simulink model "aircraft_trimLin"  (R2023a)
settings: Solver=VariableStepAuto  StartTime=0.0  StopTime=TF  RelTol=1e-3
values from neighbouring files (symbols this model uses):
  x0 = [85; 0; 0; 0; 0; 0; 0; 0.1; 0; 44.94028*pi/180; -73.09747*pi/180; 3000*0.2808]    [init.m]
undefined symbols (not defined in the file or in its folder): aircraft_6DOF_model
libraries: aerolibfltsims x2, aerolibanimutils x1
settings Model: Creator=Hegde  LastModifiedBy=Hegde

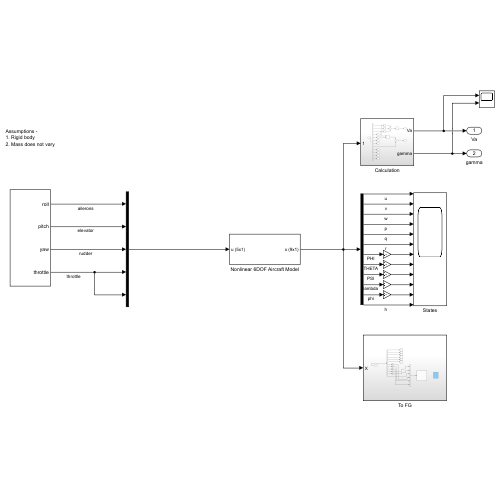
[thumbnail: Simulink's stored preview of the top-level diagram]
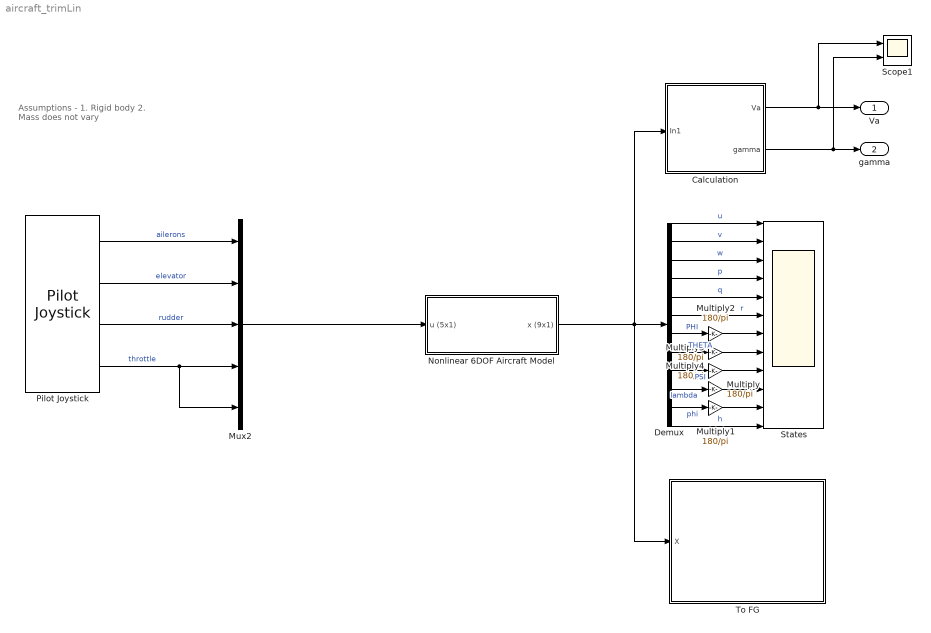
== system aircraft_trimLin ==
  note: Assumptions -
      | 1. Rigid body
      | 2. Mass does not vary
  Calculation : Subsystem
  Demux : Demux  Outputs=12
  Multiply{,1..4} (5 alike) : Gain  Gain=180/pi
  Mux2 : Mux  Inputs=5
  Nonlinear 6DOF Aircraft Model : Subsystem
  Pilot Joystick : aerolibanimutils/Pilot Joystick  JoystickID=Joystick1  OutputConfiguration=FourAxis  SampleTime=1/30
  Scope1 : Scope  NumInputPorts=2
  States : Scope  NumInputPorts=12
  To FG : Subsystem
  Va : Outport
  gamma : Outport  Port=2
  wires:
  Demux/1 -> States/1  "u"
  Demux/2 -> States/2  "v"
  Demux/3 -> States/3  "w"
  Demux/4 -> States/4  "p"
  Demux/5 -> States/5  "q"
  Demux/6 -> States/6  "r"
  Demux/7 -> Multiply2/1  "PHI"
  Demux/8 -> Multiply3/1  "THETA"
  Demux/9 -> Multiply4/1  "PSI"
  Calculation/2(gamma) -> Scope1/2, gamma/1
  Calculation/1(Va) -> Va/1, Scope1/1
  Mux2/1 -> Nonlinear 6DOF Aircraft Model/1(u (5x1))
  Pilot Joystick/1 -> Mux2/1  "ailerons"
  Pilot Joystick/2 -> Mux2/2  "elevator"
  Pilot Joystick/3 -> Mux2/3  "rudder"
  Pilot Joystick/4 -> Mux2/4, Mux2/5  "throttle"
  Demux/10 -> Multiply/1  "lambda"
  Demux/11 -> Multiply1/1  "phi"
  Demux/12 -> States/12  "h"
  Multiply/1 -> States/10
  Multiply1/1 -> States/11
  Multiply2/1 -> States/7
  Multiply3/1 -> States/8
  Multiply4/1 -> States/9
  Nonlinear 6DOF Aircraft Model/1(x (9x1)) -> To FG/1(X), Demux/1, Calculation/1(In1)

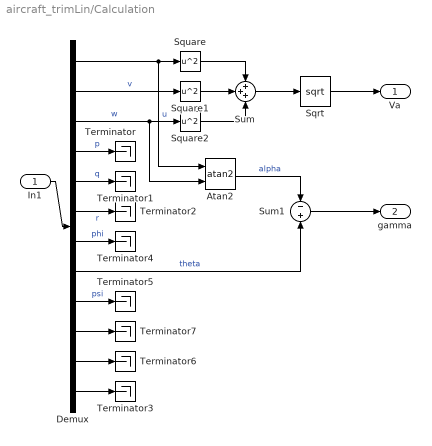
== system aircraft_trimLin/Calculation ==
  In1 : Inport
  Atan2 : Trigonometry  Operator=atan2
  Demux : Demux  Outputs=12
  Sqrt : Sqrt
  Square : Math  Operator=square
  Square1 : Math  Operator=square
  Square2 : Math  Operator=square
  Sum : Sum  Inputs=+++
  Sum1 : Sum  Inputs=-+
  Terminator{,1..7} (8 alike) : Terminator
  Va : Outport
  gamma : Outport  Port=2
  wires:
  Demux/1 -> Atan2/1, Square/1  "u"
  Square/1 -> Sum/1
  Demux/9 -> Terminator5/1  "psi"
  Demux/5 -> Terminator1/1  "q"
  Demux/3 -> Square2/1, Atan2/2  "w"
  In1/1 -> Demux/1
  Demux/2 -> Square1/1  "v"
  Demux/6 -> Terminator2/1  "r"
  Atan2/1 -> Sum1/1  "alpha"
  Demux/4 -> Terminator/1  "p"
  Sum1/1 -> gamma/1
  Square2/1 -> Sum/3
  Sum/1 -> Sqrt/1
  Demux/7 -> Terminator4/1  "phi"
  Demux/8 -> Sum1/2  "theta"
  Square1/1 -> Sum/2
  Sqrt/1 -> Va/1
  Demux/12 -> Terminator3/1
  Demux/10 -> Terminator7/1
  Demux/11 -> Terminator6/1

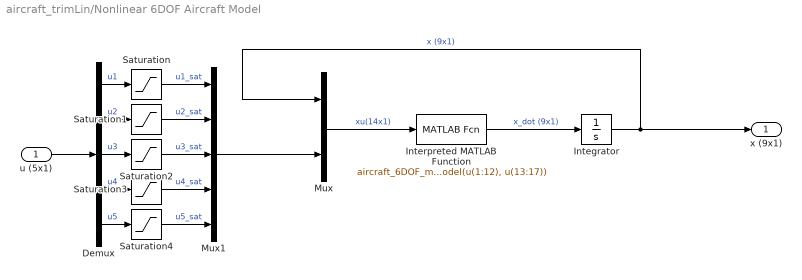
== system aircraft_trimLin/Nonlinear 6DOF Aircraft Model ==
  u (5x1) : Inport
  Demux : Demux  Outputs=5
  Integrator : Integrator  InitialCondition=x0
  Interpreted MATLAB Function : MATLABFcn  MATLABFcn=aircraft_6DOF_model(u(1:12), u(13:17))
  Mux : Mux  Inputs=2
  Mux1 : Mux  Inputs=5
  Saturation : Saturate  UpperLimit=25 * pi/180  LowerLimit=-25 * pi/180
  Saturation1 : Saturate  UpperLimit=10 * pi/180  LowerLimit=-25 * pi/180
  Saturation2 : Saturate  UpperLimit=30 * pi/180  LowerLimit=-30 * pi/180
  Saturation3 : Saturate  UpperLimit=1  LowerLimit=0
  Saturation4 : Saturate  UpperLimit=1  LowerLimit=0
  x (9x1) : Outport
  wires:
  Integrator/1 -> x (9x1)/1, Mux/1  "x (9x1)"
  Interpreted MATLAB Function/1 -> Integrator/1  "x_dot (9x1)"
  Mux/1 -> Interpreted MATLAB Function/1  "xu(14x1)"
  u (5x1)/1 -> Demux/1
  Demux/1 -> Saturation/1  "u1"
  Saturation/1 -> Mux1/1  "u1_sat"
  Demux/2 -> Saturation1/1  "u2"
  Saturation1/1 -> Mux1/2  "u2_sat"
  Demux/3 -> Saturation2/1  "u3"
  Saturation2/1 -> Mux1/3  "u3_sat"
  Demux/4 -> Saturation3/1  "u4"
  Demux/5 -> Saturation4/1  "u5"
  Saturation3/1 -> Mux1/4  "u4_sat"
  Saturation4/1 -> Mux1/5  "u5_sat"
  Mux1/1 -> Mux/2

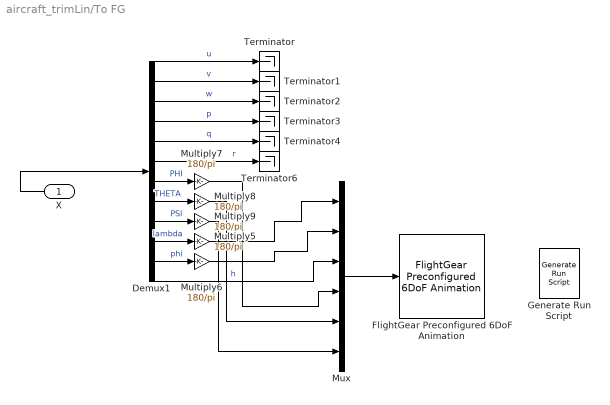
== system aircraft_trimLin/To FG ==
  X : Inport
  Demux1 : Demux  Outputs=12
  FlightGear Preconfigured 6DoF Animation : aerolibfltsims/FlightGear Preconfigured 6DoF Animation  xFlightGearVersion=v2019.1  DestinationIpAddress=127.0.0.1  DestinationPort=5502  SampleTime=1/30  packetVersion=24
  Generate Run Script : aerolibfltsims/Generate Run Script  Architecture=Default  dataFlow=Send  GeometryModelName=c172p  AirportId=KSFO  RunwayId=10L  InitialAltitude=3000*0.2808  InitialHeading=113  OffsetDistance=4.72  OffsetAzimuth=0  InstallScenery=on  DisableShaders=on  OriginAddress=127.0.0.1  DestinationPort=5502  OriginPort=5505  LocalAddress=127.0.0.1  OutputFileName=runfg.bat  FlightGearBaseDirectory=C:\Program Files\FlightGear 2024.1
  Multiply{5..9} (5 alike) : Gain  Gain=180/pi
  Mux : Mux  Inputs=6
  Terminator{,1..4,6} (6 alike) : Terminator
  wires:
  Demux1/4 -> Terminator3/1  "p"
  Demux1/10 -> Multiply5/1  "lambda"
  Demux1/7 -> Multiply7/1  "PHI"
  Multiply7/1 -> Mux/4
  Demux1/1 -> Terminator/1  "u"
  Demux1/11 -> Multiply6/1  "phi"
  Demux1/12 -> Mux/3  "h"
  Demux1/9 -> Multiply9/1  "PSI"
  Demux1/8 -> Multiply8/1  "THETA"
  Multiply5/1 -> Mux/1
  Mux/1 -> FlightGear Preconfigured 6DoF Animation/1
  Multiply9/1 -> Mux/6
  Demux1/6 -> Terminator6/1  "r"
  Multiply8/1 -> Mux/5
  Demux1/3 -> Terminator2/1  "w"
  Demux1/2 -> Terminator1/1  "v"
  Multiply6/1 -> Mux/2
  Demux1/5 -> Terminator4/1  "q"
  X/1 -> Demux1/1
